simulink model "Copy_of_alter_drum"  (R2020a)
settings: Solver=ode8  StartTime=0.0  StopTime=2  FixedStep=0.00003  RelTol=1e-3
values from neighbouring files (symbols this model uses):
  freq1 = 3    [Impedance_Learning.m]    (also in Rep.m)
  k1 = k1*(alpha^(desired_hit-hit))    [Impedance_Learning.m]    (also in Rep.m)
undefined symbols (not defined in the file or in its folder): i
libraries: simulink x2
settings Model: Creator=mojta  LastModifiedBy=mojta

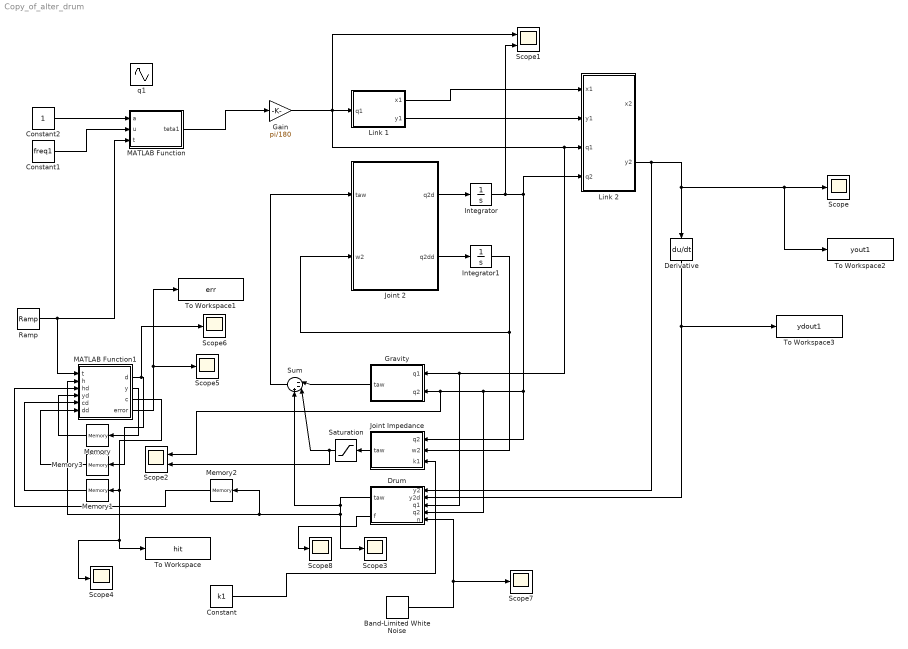
== system Copy_of_alter_drum ==
  Band-Limited White Noise : simulink/Sources/Band-Limited White Noise  Cov=[.002]  Ts=0.03  seed=[23341+10*i]
  Constant : Constant  Value=k1
  Constant1 : Constant  Value=freq1
  Constant2 : Constant
  Derivative : Derivative
  Drum : MATLAB Function  TreatAsAtomicUnit=on
  Gain : Gain  Gain=pi/180
  Gravity : MATLAB Function  TreatAsAtomicUnit=on
  Integrator : Integrator  InitialCondition=-15*pi/180
  Integrator1 : Integrator
  Joint 2 : MATLAB Function  TreatAsAtomicUnit=on
  Joint Impedance : MATLAB Function  TreatAsAtomicUnit=on
  Link 1 : MATLAB Function  TreatAsAtomicUnit=on
  Link 2 : MATLAB Function  TreatAsAtomicUnit=on
  MATLAB Function : MATLAB Function  TreatAsAtomicUnit=on
  MATLAB Function1 : MATLAB Function  TreatAsAtomicUnit=on
  Memory{,1..3} (4 alike) : Memory  InheritSampleTime=on
  Ramp : simulink/Sources/Ramp  slope=1  start=0  InitialOutput=0
  Saturation : Saturate  UpperLimit=2  LowerLimit=-2
  Scope{,3..8} (7 alike) : Scope
  Scope1 : Scope  NumInputPorts=2
  Scope2 : Scope  NumInputPorts=2
  Sum : Sum  Inputs=|--+
  To Workspace : ToWorkspace  VariableName=hit  SampleTime=-1
      settings: Save2DSignal=2-D array (concatenate along first dimension)
  To Workspace1 : ToWorkspace  VariableName=err  SampleTime=-1
      settings: Save2DSignal=2-D array (concatenate along first dimension)
  To Workspace2 : ToWorkspace  VariableName=yout1  SampleTime=-1
      settings: Save2DSignal=2-D array (concatenate along first dimension)
  To Workspace3 : ToWorkspace  VariableName=ydout1  SampleTime=-1
      settings: Save2DSignal=2-D array (concatenate along first dimension)
  q1 : Sin  Amplitude=10  Bias=30  Frequency=2*pi*3  Phase=pi/2  SampleTime=0
  wires:
  Drum/1(taw) -> Scope3/1, Memory2/1, MATLAB Function1/2(h), Sum/3
  Joint 2/2(q2dd) -> Integrator1/1
  Joint Impedance/1(taw) -> Saturation/1
  Integrator/1 -> Joint Impedance/1(q2), Drum/4(q2), Scope2/1, Gravity/2(q2), Link 2/4(q2), Scope1/2
  Gain/1 -> Scope1/1, Drum/3(q1), Gravity/1(q1), Link 2/3(q1), Link 1/1(q1)
  Sum/1 -> Joint 2/1(taw)
  Integrator1/1 -> Joint Impedance/2(w2), Joint 2/2(w2)
  Link 1/1(x1) -> Link 2/1(x1)
  Link 2/2(y2) -> Derivative/1, To Workspace2/1, Scope/1, Drum/1(y2)
  Derivative/1 -> To Workspace3/1, Drum/2(y2d)
  Link 1/2(y1) -> Link 2/2(y1)
  Gravity/1(taw) -> Sum/1
  Joint 2/1(q2d) -> Integrator/1
  Constant1/1 -> MATLAB Function/2(u)
  MATLAB Function/1(teta1) -> Gain/1
  Constant2/1 -> MATLAB Function/1(a)
  Ramp/1 -> MATLAB Function1/1(t), MATLAB Function/3(t)
  Constant/1 -> Joint Impedance/3(k1)
  MATLAB Function1/2(y) -> Memory/1
  Memory/1 -> MATLAB Function1/4(yd)
  MATLAB Function1/1(d) -> Scope6/1, Memory3/1
  MATLAB Function1/3(c) -> Scope4/1, To Workspace/1, Memory1/1
  Memory1/1 -> MATLAB Function1/5(cd)
  Memory2/1 -> MATLAB Function1/3(hd)
  Memory3/1 -> MATLAB Function1/6(dd)
  MATLAB Function1/4(error) -> Scope5/1, To Workspace1/1
  Band-Limited White Noise/1 -> Scope7/1, Drum/5(n)
  Drum/2(f) -> Scope8/1
  Saturation/1 -> Scope2/2, Sum/2

== matlab function Copy_of_alter_drum/Joint 2 ==
  data: taw input; q2d output; w2 input; q2dd output
function [q2d,q2dd] = fcn(taw,w2)

m=0.04;
L=0.4;
L2=0.3;
D2=0.1;
I=m*(3*L2^2-3*L2*L+L^2)/3;

q2d=w2;
q2dd=taw/I;

== matlab function Copy_of_alter_drum/Link 1 ==
  data: q1 input; x1 output; y1 output
function [x1,y1] = fcn(q1)

x1=0.1*cos(q1);
y1=0.1*sin(q1);

== matlab function Copy_of_alter_drum/Gravity ==
  data: q1 input; taw output; q2 input
function taw = fcn(q1,q2)

m=0.04;
g=9.8;
D2=0.1;

taw=m*g*D2*cos(q1+q2);

== matlab function Copy_of_alter_drum/Link 2 ==
  data: x1 input; y1 input; q1 input; x2 output; q2 input; y2 output
function [x2,y2] = fcn(x1,y1,q1,q2)

x2=x1+0.3*cos(q1+q2);
y2=y1+0.3*sin(q1+q2);

== matlab function Copy_of_alter_drum/Joint Impedance ==
  data: q2 input; taw output; w2 input; k1 input
function taw = fcn(q2,w2,k1)

border=-15*pi/180;

% 
% k2=200;
% d1=0.00001;
% d2=8;
% 
% if q2>border
%     taw=k1*(q2-border)+d1*w2;
% else
%     taw=k2*(q2-border)+d2*w2;
% end

b=.01;

taw=k1*(q2-border)+b*w2;

if q2<border
    taw=taw*50;
end

== matlab function Copy_of_alter_drum/Drum ==
  data: y2 input; taw output; y2d input; q1 input; q2 input; n input; f output
function [taw,f] = fcn(y2,y2d,q1,q2,n)

k=20000;
d=.1;

height=0.07;

if y2<-height
    f=(k*(y2+height)+d*y2d)*(1+n);
else
    f=0;
end

taw=-f*0.3*cos(q1+q2);

== matlab function Copy_of_alter_drum/MATLAB Function ==
  data: a input; u input; teta1 output; t input
function teta1 = fcn(a,u,t)

Amp=15;
Bias=10;



Freq=2*pi*u;
Phase=pi/2;
teta1 = Amp*sin(Freq*t+Phase) + Bias;

== matlab function Copy_of_alter_drum/MATLAB Function1 ==
  data: d output; t input; h input; hd input; y output; yd input; cd input; c output; dd input; error output
function [d,y,c,error]  = fcn(t,h,hd,yd,cd,dd)


if h>2
    y=t;
    d=y-yd;
else
    y=yd;
    d=dd;
end
error=abs(d-dd);

if h>.01 && hd==0
    c=cd+1;
else
    c=cd;
end
